simulink library "AuxEq_Lib"  (Simulink 7.5)
settings: Solver=ode45  SolverMode=SingleTasking  StartTime=0.0  StopTime=10.0  RelTol=1e-3
values from neighbouring files (symbols this model uses):
  AC = FASER_config    [UAV_config.m]    (also in UAV_modelconfig.mat = )
  TrimCondition =     [UAV_trimcondition.mat]
libraries: aerolibasang x2, simulink x2, Navigation_Lib x1, aerolib6dofsys x1
settings Model: Creator=Paul Freeman  LastModifiedBy=Andrei

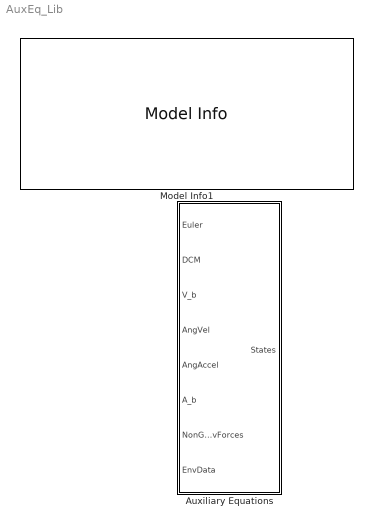
== system AuxEq_Lib ==
  Auxiliary Equations : Subsystem
  Model Info1 : simulink/Model-Wide Utilities/Model Info  SystemSampleTime=-1  InitialBlockCM=None  BlockCM=None  Frame=on  DisplayStringWithTags=|  HorizontalTextAlignment=Left  LeftAlignmentValue=0.02  SourceBlockDiagram=AuxEq_Lib  TagMaxNumber=20
      | MODEL INFORMATION
      | Auxiliary Equations Library
      | 
      | University of Minnesota
      | Aerospace Engineering and Mechanics
      | Copyright 2011 Regents of the University of Minnesota. All rights reserved.
      | 
      | == SVN Info ==
      | %<ModelVersion>
      | Last modified by %<LastModifiedBy> on %<LastModificationDate>

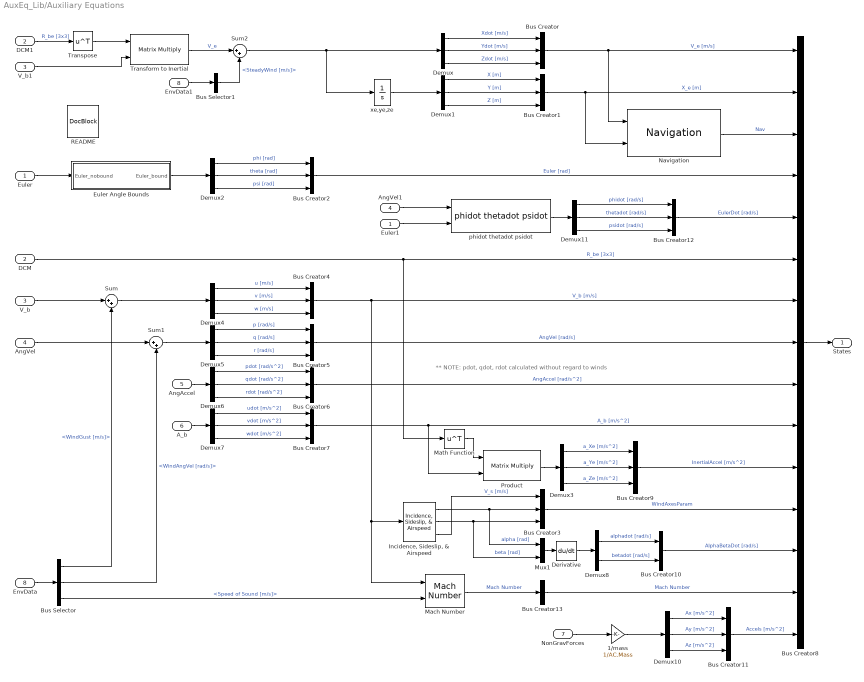
== system AuxEq_Lib/Auxiliary Equations ==
  note: ** NOTE: pdot, qdot, rdot calculated without regard to winds
  Euler : Inport  OutDataType=sfix(16)  OutScaling=2^0
  DCM : Inport  Port=2  OutDataType=sfix(16)  OutScaling=2^0
  V_b : Inport  Port=3  OutDataType=sfix(16)  OutScaling=2^0
  AngVel : Inport  Port=4  OutDataType=sfix(16)  OutScaling=2^0
  AngAccel : Inport  Port=5  OutDataType=sfix(16)  OutScaling=2^0
  A_b : Inport  Port=6  OutDataType=sfix(16)  OutScaling=2^0
  NonGravForces : Inport  Port=7  OutDataType=sfix(16)  OutScaling=2^0
  EnvData : Inport  Port=8  OutDataType=sfix(16)  OutScaling=2^0
  1/mass : Gain  Gain=1/AC.Mass  ParameterDataType=fixdt(1, 16)  ParameterScaling=2^0  OutDataType=fixdt(1, 16)  OutScaling=2^0
  AngVel1 : InportShadow  Port=4  OutDataType=sfix(16)  OutScaling=2^0
  Bus Creator{,1..7,9,11..12} (11 alike) : BusCreator  Inputs=3
  Bus Creator10 : BusCreator  Inputs=2
  Bus Creator13 : BusCreator  Inputs=1
  Bus Creator8 : BusCreator  Inputs=15
  Bus Selector : BusSelector  OutputSignals=WindGust [m/s],WindAngVel [rad/s],Speed of Sound [m/s]
  Bus Selector1 : BusSelector  OutputSignals=SteadyWind [m/s]
  DCM1 : InportShadow  Port=2  OutDataType=sfix(16)  OutScaling=2^0
  Demux{,1..7,10..11} (10 alike) : Demux  Outputs=3
  Demux8 : Demux  Outputs=2
  Derivative : Derivative
  EnvData1 : InportShadow  Port=8  OutDataType=sfix(16)  OutScaling=2^0
  Euler Angle Bounds : Subsystem
  Euler1 : InportShadow  Port=1  OutDataType=sfix(16)  OutScaling=2^0
  "Incidence, Sideslip, & Airspeed" : aerolibasang/Incidence, Sideslip, & Airspeed  SystemSampleTime=-1
  Mach Number : aerolibasang/Mach Number  SystemSampleTime=-1
  Math Function : Math  Operator=transpose  OutDataType=fixdt(1, 16)  OutScaling=2^0  SaturateOnIntegerOverflow=on
  Mux1 : Mux  Inputs=2
  Navigation : Navigation_Lib/Navigation  Description=|  SystemSampleTime=-1
      | This model produces the followng navigation data for the UAV flight:
      |                                                                     
      | * Geodetic Latitude                                                 
      | * Geodetic Longitude                                                
      | * Geodetic Altitude                                                 
      | * Altitude above Mean Sea Level                                     
      | * Gravitational acceleration vector
  Product : Product  Multiplication=Matrix(*)  OutDataType=fixdt(1, 16)  OutScaling=2^0  RndMeth=Zero
  README : simulink/Model-Wide Utilities/DocBlock  SystemSampleTime=-1  DocumentType=Text
      content=|
      | Auxiliary Equations
      |
      | This block computes other relevant variables (such as angle of attack,
      | indicated airspeed, etc) from state data. Part of this block is simply to
      | assign signals name and create the States bus.
      |
      | Working from the top of the block downwards:
      |
      | The inertial velocity, V_e, is computed by using the Direction Cosine
      | Matrix (DCM) to transform the body-axis velocities (u,v,w) to the
      | inertial frame. The steady state winds are then added, and the result is
      | V_e. This is integrated to obtain the inertial position, X_e.  The
      | initial condition of the X_e integrator is set by
      | TrimCondition.InertialIni. V_e and X_e are inputs to the Navigation
      | block- see that blocks README for details.
      |
      | Euler angles are bounded by +\- [pi/2, pi, 2*pi] respectively. The time
      | derivatives of the Euler angles are computed using the body-axis rates
      | and the Euler angles.
      |
      | The DCM is included in the States bus as "R_be [3x3]".
      |
      | Body axis velocites and rates, and their derivatives are included. The
      | unsteady (turbulence and gusts) winds are added to the body axis
      | velocities and rates.
      |
      | Inertial accelerations are computed by transforming the body-axis
      | accelerations with the DCM. This step is simplified since we are using a
      | non-rotating Earth.
      |
      | WindAxesParam is the true airspeed, angle of attack, and sideslip angle.
      | The derivatives of alpha and beta are computed using a deriative block.
      | Mach number is simply the ratio between true airspeed and the speed of
      | sound.
      |
      | Accels [m/s^2] is what an accelerometer would read onboard the aircraft.
      |
      | *Note on winds: dividing the wind components into steady and unsteady
      | components is necessary because we do not use an intermediate atmospheric
      | reference frame to account for the motion of the air mass relative to the
      | Earth. We can approximate the physical effects of wind without an
      | additional reference frame by splitting the wind into steady and unsteady
      | components, where the steady component is added to the inertial
      | velocities and the unsteady component is added to the body-axis
      | velocities allows us to
  Sum : Sum  Inputs=|++  OutDataType=sfix(16)  OutScaling=2^0
  Sum1 : Sum  Inputs=|++  OutDataType=sfix(16)  OutScaling=2^0
  Sum2 : Sum  Inputs=|++  OutDataType=sfix(16)  OutScaling=2^0
  Transform to Inertial : Product  Multiplication=Matrix(*)  OutDataType=fixdt(1, 16)  OutScaling=2^0  RndMeth=Zero
  Transpose : Math  Operator=transpose  OutDataType=sfix(16)  OutScaling=2^0  SaturateOnIntegerOverflow=on
  V_b1 : InportShadow  Port=3  OutDataType=sfix(16)  OutScaling=2^0
  phidot thetadot psidot : aerolib6dofsys/DCM & Euler Angles (Euler)/phidot thetadot psidot  SystemSampleTime=-1
  xe,ye,ze : Integrator  InitialCondition=TrimCondition.InertialIni
  States : Outport  OutDataType=sfix(16)  OutScaling=2^0
  wires:
  Euler Angle Bounds/1(Euler_bound) -> Demux2/1
  Euler/1 -> Euler Angle Bounds/1(Euler_nobound)
  V_b1/1 -> Transform to Inertial/2
  xe,ye,ze/1 -> Demux1/1
  Sum2/1 -> xe,ye,ze/1, Demux/1
  Bus Selector1/1 -> Sum2/2  "<SteadyWind [m/s]>"
  Transform to Inertial/1 -> Sum2/1  "V_e"
  EnvData1/1 -> Bus Selector1/1
  DCM1/1 -> Transpose/1  "R_be [3x3]"
  Transpose/1 -> Transform to Inertial/1
  phidot thetadot psidot/1 -> Demux11/1
  Bus Creator12/1 -> Bus Creator8/5  "EulerDot [rad/s]"
  Demux11/1 -> Bus Creator12/1  "phidot [rad/s]"
  Demux11/2 -> Bus Creator12/2  "thetadot [rad/s]"
  Demux11/3 -> Bus Creator12/3  "psidot [rad/s]"
  Demux10/3 -> Bus Creator11/3  "Az [m/s^2]"
  Demux10/2 -> Bus Creator11/2  "Ay [m/s^2]"
  Demux10/1 -> Bus Creator11/1  "Ax [m/s^2]"
  1/mass/1 -> Demux10/1
  NonGravForces/1 -> 1/mass/1
  Bus Creator/1 -> Navigation/1, Bus Creator8/1  "V_e [m/s]"
  Demux/1 -> Bus Creator/1  "Xdot [m/s]"
  Demux/2 -> Bus Creator/2  "Ydot [m/s]"
  Demux/3 -> Bus Creator/3  "Zdot [m/s]"
  Bus Creator1/1 -> Navigation/2, Bus Creator8/2  "X_e [m]"
  Demux1/1 -> Bus Creator1/1  "X [m]"
  Demux1/2 -> Bus Creator1/2  "Y [m]"
  Demux1/3 -> Bus Creator1/3  "Z [m]"
  Bus Creator2/1 -> Bus Creator8/4  "Euler [rad]"
  Demux2/1 -> Bus Creator2/1  "phi [rad]"
  Demux2/2 -> Bus Creator2/2  "theta [rad]"
  Demux2/3 -> Bus Creator2/3  "psi [rad]"
  DCM/1 -> Math Function/1, Bus Creator8/6  "R_be [3x3]"
  Bus Creator4/1 -> Bus Creator8/7, "Incidence, Sideslip, & Airspeed"/1, Mach Number/1  "V_b [m/s]"
  Demux4/1 -> Bus Creator4/1  "u [m/s]"
  Demux4/2 -> Bus Creator4/2  "v [m/s]"
  Demux4/3 -> Bus Creator4/3  "w [m/s]"
  Bus Creator5/1 -> Bus Creator8/8  "AngVel [rad/s]"
  Demux5/1 -> Bus Creator5/1  "p [rad/s]"
  Demux5/2 -> Bus Creator5/2  "q [rad/s]"
  Demux5/3 -> Bus Creator5/3  "r [rad/s]"
  Bus Creator6/1 -> Bus Creator8/9  "AngAccel [rad/s^2]"
  Demux6/1 -> Bus Creator6/1  "pdot [rad/s^2]"
  Demux6/2 -> Bus Creator6/2  "qdot [rad/s^2]"
  Demux6/3 -> Bus Creator6/3  "rdot [rad/s^2]"
  AngAccel/1 -> Demux6/1
  Bus Creator7/1 -> Product/2, Bus Creator8/10  "A_b [m/s^2]"
  Demux7/1 -> Bus Creator7/1  "udot [m/s^2]"
  Demux7/2 -> Bus Creator7/2  "vdot [m/s^2]"
  Demux7/3 -> Bus Creator7/3  "wdot [m/s^2]"
  A_b/1 -> Demux7/1
  Bus Creator3/1 -> Bus Creator8/12  "WindAxesParam"
  Bus Creator13/1 -> Bus Creator8/14  "Mach Number"
  EnvData/1 -> Bus Selector/1
  Bus Selector/3 -> Mach Number/2  "<Speed of Sound [m/s]>"
  Sum1/1 -> Demux5/1
  Sum/1 -> Demux4/1
  AngVel/1 -> Sum1/1
  V_b/1 -> Sum/1
  Math Function/1 -> Product/1
  Product/1 -> Demux3/1
  Demux3/1 -> Bus Creator9/1  "a_Xe [m/s^2]"
  Demux3/3 -> Bus Creator9/3  "a_Ze [m/s^2]"
  Demux3/2 -> Bus Creator9/2  "a_Ye [m/s^2]"
  Bus Creator9/1 -> Bus Creator8/11  "InertialAccel [m/s^2]"
  Bus Selector/2 -> Sum1/2  "<WindAngVel [rad/s]>"
  Bus Selector/1 -> Sum/2  "<WindGust [m/s]>"
  AngVel1/1 -> phidot thetadot psidot/1
  Euler1/1 -> phidot thetadot psidot/2
  Bus Creator11/1 -> Bus Creator8/15  "Accels [m/s^2]"
  Navigation/1 -> Bus Creator8/3  "Nav"
  Bus Creator8/1 -> States/1
  "Incidence, Sideslip, & Airspeed"/1 -> Bus Creator3/2, Mux1/1  "alpha [rad]"
  "Incidence, Sideslip, & Airspeed"/2 -> Bus Creator3/3, Mux1/2  "beta [rad]"
  "Incidence, Sideslip, & Airspeed"/3 -> Bus Creator3/1  "V_s [m/s]"
  Mux1/1 -> Derivative/1
  Derivative/1 -> Demux8/1
  Bus Creator10/1 -> Bus Creator8/13  "AlphaBetaDot [rad/s]"
  Demux8/1 -> Bus Creator10/1  "alphadot [rad/s]"
  Demux8/2 -> Bus Creator10/2  "betadot [rad/s]"
  Mach Number/1 -> Bus Creator13/1  "Mach Number"

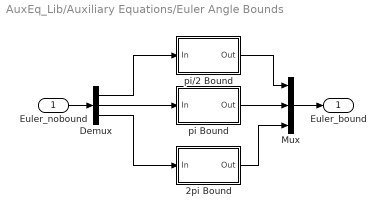
== system AuxEq_Lib/Auxiliary Equations/Euler Angle Bounds ==
  Euler_nobound : Inport
  2pi Bound : Subsystem
  Demux : Demux  Outputs=3
  Mux : Mux  Inputs=3
  pi Bound : Subsystem
  pi/2 Bound : Subsystem
  Euler_bound : Outport
  wires:
  pi Bound/1(Out) -> Mux/2
  pi/2 Bound/1(Out) -> Mux/1
  Mux/1 -> Euler_bound/1
  Euler_nobound/1 -> Demux/1
  Demux/1 -> pi/2 Bound/1(In)
  Demux/2 -> pi Bound/1(In)
  Demux/3 -> 2pi Bound/1(In)
  2pi Bound/1(Out) -> Mux/3

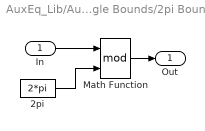
== system AuxEq_Lib/Auxiliary Equations/Euler Angle Bounds/2pi Bound ==
  In : Inport  OutDataType=sfix(16)  OutScaling=2^0
  2pi : Constant  Value=2*pi  OutDataType=sfix(16)  OutScaling=2^0
  Math Function : Math  Operator=mod  SaturateOnIntegerOverflow=on
  Out : Outport
  wires:
  Math Function/1 -> Out/1
  2pi/1 -> Math Function/2
  In/1 -> Math Function/1

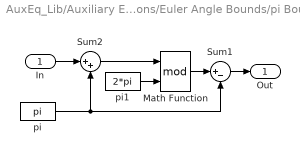
== system AuxEq_Lib/Auxiliary Equations/Euler Angle Bounds/pi Bound ==
  In : Inport  OutDataType=sfix(16)  OutScaling=2^0
  Math Function : Math  Operator=mod  SaturateOnIntegerOverflow=on
  Sum1 : Sum  Inputs=|+-  OutDataType=sfix(16)  OutScaling=2^0  SaturateOnIntegerOverflow=on  InputSameDT=on  OutDataTypeStr=Inherit: Same as first input
  Sum2 : Sum  Inputs=|++  OutDataType=sfix(16)  OutScaling=2^0  SaturateOnIntegerOverflow=on  InputSameDT=on  OutDataTypeStr=Inherit: Same as first input
  pi : Constant  Value=pi  OutDataType=sfix(16)  OutScaling=2^0
  pi1 : Constant  Value=2*pi  OutDataType=sfix(16)  OutScaling=2^0
  Out : Outport
  wires:
  Math Function/1 -> Sum1/1
  pi1/1 -> Math Function/2
  In/1 -> Sum2/1
  Sum2/1 -> Math Function/1
  pi/1 -> Sum2/2, Sum1/2
  Sum1/1 -> Out/1

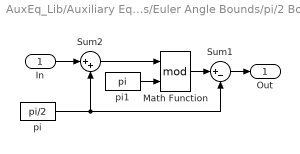
== system AuxEq_Lib/Auxiliary Equations/Euler Angle Bounds/pi/2 Bound ==
  In : Inport  OutDataType=sfix(16)  OutScaling=2^0
  Math Function : Math  Operator=mod  SaturateOnIntegerOverflow=on
  Sum1 : Sum  Inputs=|+-  OutDataType=sfix(16)  OutScaling=2^0  SaturateOnIntegerOverflow=on  InputSameDT=on  OutDataTypeStr=Inherit: Same as first input
  Sum2 : Sum  Inputs=|++  OutDataType=sfix(16)  OutScaling=2^0  SaturateOnIntegerOverflow=on  InputSameDT=on  OutDataTypeStr=Inherit: Same as first input
  pi : Constant  Value=pi/2  OutDataType=sfix(16)  OutScaling=2^0
  pi1 : Constant  Value=pi  OutDataType=sfix(16)  OutScaling=2^0
  Out : Outport
  wires:
  Sum1/1 -> Out/1
  pi/1 -> Sum1/2, Sum2/2
  Sum2/1 -> Math Function/1
  In/1 -> Sum2/1
  pi1/1 -> Math Function/2
  Math Function/1 -> Sum1/1
